simulink library "AeroCoefficientLibrary"  (R2024a)
settings: Solver=VariableStepAuto  StartTime=0.0  StopTime=10.0  RelTol=1e-3
undefined symbols (not defined in the file): alphaBkpts_nd, betaBkpts_nd, CL, CX, dLdRud, elevBkpts_nd
settings Model: Creator=jerem  LastModifiedBy=jerem

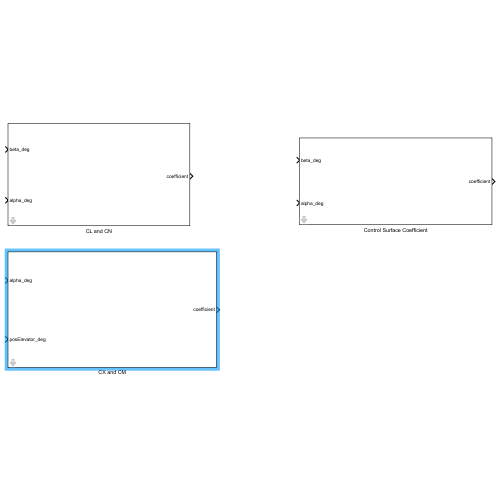
[thumbnail: Simulink's stored preview of the top-level diagram]
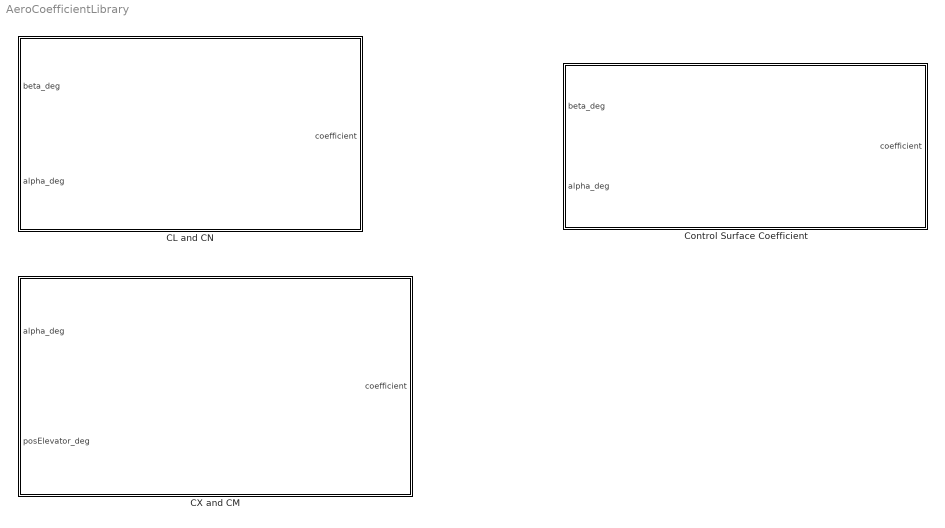
== system AeroCoefficientLibrary ==
  CL and CN : Subsystem  mask{aeroData=CL, betaBkpts_nd=betaBkpts_nd, alphaBkpts_nd=alphaBkpts_nd}
      mask prompts: aeroData "TableData"; betaBkpts_nd "Beta Bkpts"; alphaBkpts_nd "Alpha Bkpts"
  CX and CM : Subsystem  mask{aeroData=CX, alphaBkpts_nd=alphaBkpts_nd, elevBkpts_nd=elevBkpts_nd}
      mask prompts: aeroData "Table Data"; alphaBkpts_nd "Alpha Bkpts"; elevBkpts_nd "Elevator Bkpts"
  Control Surface Coefficient : Subsystem  mask{aeroData=dLdRud, betaBkpts_nd=betaBkpts_nd, alphaBkpts_nd=alphaBkpts_nd}
      mask prompts: aeroData "Table Data"; betaBkpts_nd "Beta Bkpts"; alphaBkpts_nd "Alpha Bkpts"

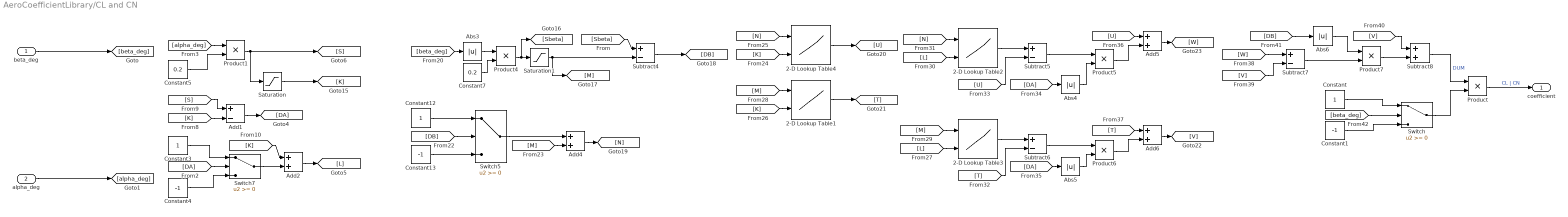
== system AeroCoefficientLibrary/CL and CN ==
  beta_deg : Inport
  alpha_deg : Inport  Port=2
  2-D Lookup Table{1..4} (4 alike) : Lookup_n-D  BreakpointsForDimension1=betaBkpts_nd  BreakpointsForDimension2=alphaBkpts_nd  Table=aeroData  ExtrapMethod=Clip  DiagnosticForOutOfRangeInput=Warning  InternalRulePriority=Speed  RndMeth=Simplest
      settings: InputPortMap=u0,u1
  Abs{3..6} (4 alike) : Abs  SaturateOnIntegerOverflow=off
  Add1 : Sum  Inputs=+-
  Add{2,4..6} (4 alike) : Sum
  Constant : Constant
  Constant1 : Constant  Value=-1
  Constant12 : Constant
  Constant13 : Constant  Value=-1
  Constant3 : Constant
  Constant4 : Constant  Value=-1
  Constant5 : Constant  Value=0.2
  Constant7 : Constant  Value=0.2
  Product{,1,4..7} (6 alike) : Product
  Saturation : Saturate  UpperLimit=8  LowerLimit=-1
  Saturation1 : Saturate  UpperLimit=5  LowerLimit=1
  Subtract{4..7} (4 alike) : Sum  Inputs=+-
  Subtract8 : Sum
  Switch : Switch  SaturateOnIntegerOverflow=off  InputSameDT=off
  Switch5 : Switch  SaturateOnIntegerOverflow=off  InputSameDT=off
  Switch7 : Switch  SaturateOnIntegerOverflow=off  InputSameDT=off
  coefficient : Outport
  wires:
  Saturation1/1 -> Subtract4/2, [M]
  Subtract7/1 -> Product7/2
  Constant13/1 -> Switch5/3
  Abs4/1 -> Product5/2
  2-D Lookup Table3/1 -> Subtract6/1
  [DB] -> Switch5/2
  [U] -> Subtract5/2
  Subtract8/1 -> Product/1  "DUM"
  Constant12/1 -> Switch5/1
  Abs5/1 -> Product6/2
  Subtract4/1 -> [DB]
  [Sbeta] -> Subtract4/1
  [T] -> Add6/1
  [T] -> Subtract6/2
  Product4/1 -> Saturation1/1, [Sbeta]
  [M] -> 2-D Lookup Table3/1
  [beta_deg] -> Abs3/1
  Product6/1 -> Add6/2
  2-D Lookup Table1/1 -> [T]
  [K] -> 2-D Lookup Table4/2
  [V] -> Subtract8/1
  [W] -> Subtract7/1
  [N] -> 2-D Lookup Table4/1
  [DA] -> Abs4/1
  Subtract6/1 -> Product6/1
  2-D Lookup Table2/1 -> Subtract5/1
  Abs3/1 -> Product4/1
  Switch5/1 -> Add4/1
  [M] -> 2-D Lookup Table1/1
  Product7/1 -> Subtract8/2
  Add4/1 -> [N]
  2-D Lookup Table4/1 -> [U]
  [M] -> Add4/2
  [DA] -> Abs5/1
  [L] -> 2-D Lookup Table3/2
  [U] -> Add5/1
  [N] -> 2-D Lookup Table2/1
  Product5/1 -> Add5/2
  Add5/1 -> [W]
  [K] -> 2-D Lookup Table1/2
  [V] -> Subtract7/2
  [DB] -> Abs6/1
  Add6/1 -> [V]
  Constant7/1 -> Product4/2
  Abs6/1 -> Product7/1
  [L] -> 2-D Lookup Table2/2
  Subtract5/1 -> Product5/1
  Product/1 -> coefficient/1  "CL | CN"
  beta_deg/1 -> [beta_deg]
  alpha_deg/1 -> [alpha_deg]
  Constant3/1 -> Switch7/1
  [DA] -> Switch7/2
  Product1/1 -> Saturation/1, [S]
  Saturation/1 -> [K]
  Add1/1 -> [DA]
  Constant4/1 -> Switch7/3
  [alpha_deg] -> Product1/1
  [S] -> Add1/1
  Add2/1 -> [L]
  Constant5/1 -> Product1/2
  [K] -> Add1/2
  Switch7/1 -> Add2/2
  [K] -> Add2/1
  [beta_deg] -> Switch/2
  Constant/1 -> Switch/1
  Constant1/1 -> Switch/3
  Switch/1 -> Product/2

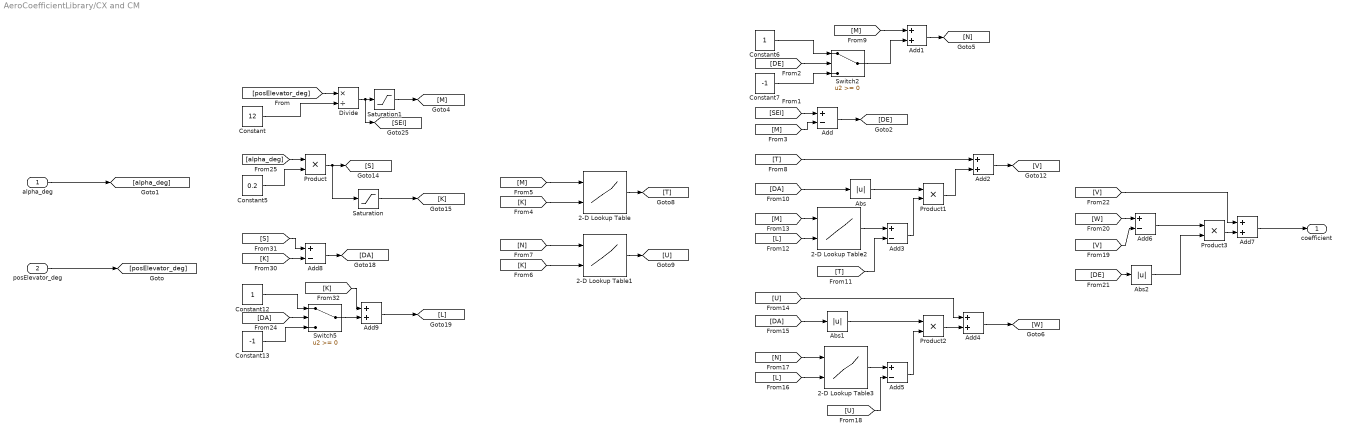
== system AeroCoefficientLibrary/CX and CM ==
  alpha_deg : Inport
  posElevator_deg : Inport  Port=2
  2-D Lookup Table{,1..3} (4 alike) : Lookup_n-D  BreakpointsForDimension1=elevBkpts_nd  BreakpointsForDimension2=alphaBkpts_nd  Table=aeroData  ExtrapMethod=Clip  DiagnosticForOutOfRangeInput=Warning  InternalRulePriority=Speed  RndMeth=Simplest
      settings: InputPortMap=u0,u1
  Abs : Abs  SaturateOnIntegerOverflow=off
  Abs1 : Abs  SaturateOnIntegerOverflow=off
  Abs2 : Abs  SaturateOnIntegerOverflow=off
  Add{,3,5..6,8} (5 alike) : Sum  Inputs=+-
  Add{1..2,4,7,9} (5 alike) : Sum
  Constant : Constant  Value=12
  Constant12 : Constant
  Constant13 : Constant  Value=-1
  Constant5 : Constant  Value=0.2
  Constant6 : Constant
  Constant7 : Constant  Value=-1
  Divide : Product  Inputs=*/
  Product{,1..3} (4 alike) : Product
  Saturation : Saturate  UpperLimit=8  LowerLimit=-1
  Saturation1 : Saturate  UpperLimit=1  LowerLimit=-1
  Switch2 : Switch  SaturateOnIntegerOverflow=off  InputSameDT=off
  Switch5 : Switch  SaturateOnIntegerOverflow=off  InputSameDT=off
  coefficient : Outport
  wires:
  Product3/1 -> Add7/2
  Add1/1 -> [N]
  Product2/1 -> Add4/2
  Constant6/1 -> Switch2/1
  Add3/1 -> Product1/2
  [DA] -> Abs/1
  Add6/1 -> Product3/1
  [DE] -> Abs2/1
  Switch2/1 -> Add1/2
  [DA] -> Abs1/1
  Product1/1 -> Add2/2
  [posElevator_deg] -> Divide/1
  Add7/1 -> coefficient/1
  Add4/1 -> [W]
  [DE] -> Switch2/2
  [V] -> Add7/1
  Abs2/1 -> Product3/2
  Constant7/1 -> Switch2/3
  [V] -> Add6/2
  [W] -> Add6/1
  [M] -> 2-D Lookup Table/1
  [L] -> 2-D Lookup Table3/2
  Abs1/1 -> Product2/1
  [N] -> 2-D Lookup Table1/1
  [N] -> 2-D Lookup Table3/1
  [K] -> 2-D Lookup Table/2
  [SEl] -> Add/1
  2-D Lookup Table2/1 -> Add3/1
  2-D Lookup Table1/1 -> [U]
  Abs/1 -> Product1/1
  2-D Lookup Table/1 -> [T]
  [M] -> 2-D Lookup Table2/1
  [T] -> Add3/2
  [M] -> Add/2
  [M] -> Add1/1
  [K] -> 2-D Lookup Table1/2
  [L] -> 2-D Lookup Table2/2
  Add/1 -> [DE]
  [T] -> Add2/1
  [U] -> Add5/2
  Add5/1 -> Product2/2
  Constant/1 -> Divide/2
  [U] -> Add4/1
  2-D Lookup Table3/1 -> Add5/1
  Add2/1 -> [V]
  Saturation1/1 -> [M]
  posElevator_deg/1 -> [posElevator_deg]
  alpha_deg/1 -> [alpha_deg]
  [alpha_deg] -> Product/1
  Constant13/1 -> Switch5/3
  Add9/1 -> [L]
  Add8/1 -> [DA]
  [DA] -> Switch5/2
  Constant12/1 -> Switch5/1
  Product/1 -> Saturation/1, [S]
  [K] -> Add8/2
  Constant5/1 -> Product/2
  Switch5/1 -> Add9/2
  [K] -> Add9/1
  [S] -> Add8/1
  Divide/1 -> [SEl], Saturation1/1
  Saturation/1 -> [K]

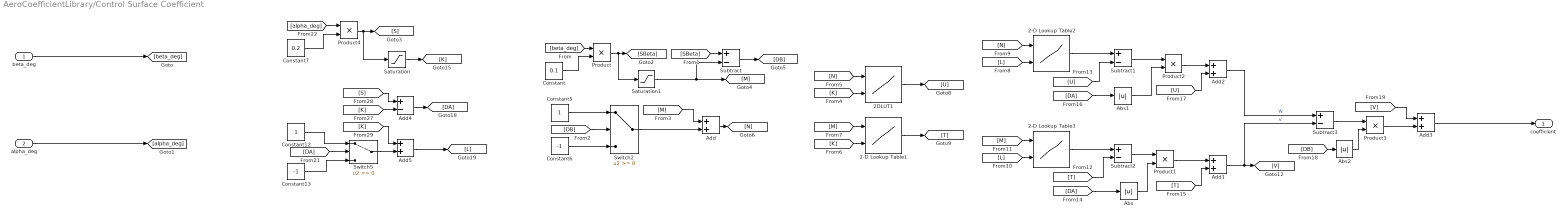
== system AeroCoefficientLibrary/Control Surface Coefficient ==
  beta_deg : Inport
  alpha_deg : Inport  Port=2
  2-D Lookup Table1 : Lookup_n-D  BreakpointsForDimension1=betaBkpts_nd  BreakpointsForDimension2=alphaBkpts_nd  Table=aeroData  ExtrapMethod=Clip  DiagnosticForOutOfRangeInput=Warning  InternalRulePriority=Speed  RndMeth=Simplest
      settings: InputPortMap=u0,u1
  2-D Lookup Table2 : Lookup_n-D  BreakpointsForDimension1=betaBkpts_nd  BreakpointsForDimension2=alphaBkpts_nd  Table=aeroData  ExtrapMethod=Clip  DiagnosticForOutOfRangeInput=Warning  InternalRulePriority=Speed  RndMeth=Simplest
      settings: InputPortMap=u0,u1
  2-D Lookup Table3 : Lookup_n-D  BreakpointsForDimension1=betaBkpts_nd  BreakpointsForDimension2=alphaBkpts_nd  Table=aeroData  ExtrapMethod=Clip  DiagnosticForOutOfRangeInput=Warning  InternalRulePriority=Speed  RndMeth=Simplest
      settings: InputPortMap=u0,u1
  2DLUT1 : Lookup_n-D  BreakpointsForDimension1=betaBkpts_nd  BreakpointsForDimension2=alphaBkpts_nd  Table=aeroData  ExtrapMethod=Clip  DiagnosticForOutOfRangeInput=Warning  InternalRulePriority=Speed  RndMeth=Simplest
      settings: InputPortMap=u0,u1
  Abs : Abs  SaturateOnIntegerOverflow=off
  Abs1 : Abs  SaturateOnIntegerOverflow=off
  Abs2 : Abs  SaturateOnIntegerOverflow=off
  Add{,1..3,5} (5 alike) : Sum
  Add4 : Sum  Inputs=+-
  Constant : Constant  Value=0.1
  Constant12 : Constant
  Constant13 : Constant  Value=-1
  Constant5 : Constant
  Constant6 : Constant  Value=-1
  Constant7 : Constant  Value=0.2
  Product{,1..4} (5 alike) : Product
  Saturation : Saturate  UpperLimit=8  LowerLimit=-1
  Saturation1 : Saturate  UpperLimit=2  LowerLimit=-2  LinearizeAsGain=off
  Subtract{,1..3} (4 alike) : Sum  Inputs=+-
  Switch2 : Switch  SaturateOnIntegerOverflow=off  InputSameDT=off
  Switch5 : Switch  SaturateOnIntegerOverflow=off  InputSameDT=off
  coefficient : Outport
  wires:
  Add3/1 -> coefficient/1
  beta_deg/1 -> [beta_deg]
  [K] -> Add5/1
  Switch5/1 -> Add5/2
  Constant7/1 -> Product4/2
  [K] -> Add4/2
  [S] -> Add4/1
  Product4/1 -> Saturation/1, [S]
  Saturation/1 -> [K]
  Constant12/1 -> Switch5/1
  [DA] -> Switch5/2
  Add4/1 -> [DA]
  Add5/1 -> [L]
  alpha_deg/1 -> [alpha_deg]
  [alpha_deg] -> Product4/1
  Constant13/1 -> Switch5/3
  Subtract1/1 -> Product2/1
  [DB] -> Abs2/1
  2DLUT1/1 -> [U]
  [T] -> Subtract2/2
  [DA] -> Abs/1
  Abs1/1 -> Product2/2
  Product3/1 -> Add3/2
  [U] -> Subtract1/2
  [L] -> 2-D Lookup Table2/2
  2-D Lookup Table2/1 -> Subtract1/1
  [U] -> Add2/2
  [T] -> Add1/2
  [N] -> 2DLUT1/1
  [DB] -> Switch2/2
  2-D Lookup Table1/1 -> [T]
  Subtract/1 -> [DB]
  Saturation1/1 -> [M], Subtract/2
  Add2/1 -> Subtract3/1  "W"
  Abs2/1 -> Product3/2
  [M] -> Add/1
  Constant/1 -> Product/2
  [SBeta] -> Subtract/1
  Constant5/1 -> Switch2/1
  Add1/1 -> Subtract3/2, [V]  "V"
  Switch2/1 -> Add/2
  Product1/1 -> Add1/1
  [DA] -> Abs1/1
  Subtract2/1 -> Product1/1
  Product/1 -> Saturation1/1, [SBeta]
  2-D Lookup Table3/1 -> Subtract2/1
  [K] -> 2-D Lookup Table1/2
  Constant6/1 -> Switch2/3
  [beta_deg] -> Product/1
  Abs/1 -> Product1/2
  [M] -> 2-D Lookup Table3/1
  Product2/1 -> Add2/1
  [V] -> Add3/1
  [L] -> 2-D Lookup Table3/2
  Subtract3/1 -> Product3/1
  Add/1 -> [N]
  [N] -> 2-D Lookup Table2/1
  [M] -> 2-D Lookup Table1/1
  [K] -> 2DLUT1/2
